simulink model "Vdc_Controller"  (R2022a)
settings: Solver=FixedStepAuto  StartTime=0.0  StopTime=TsimTime  FixedStep=Ts  MaxStep=Tsim*100  RelTol=1e-5
undefined symbols (not defined in the file): Avdc, Bvdc, IbuckSaturation, Kiv, Kpv, Ktv, Rdc, Ts
libraries: simulink x1
settings Model: Creator=MasterGnome  LastModifiedBy=MasterGnome
settings SolverCC: ZeroCrossAlgorithm=Adaptive
settings DataIOCC: SaveOutput=off  SaveTime=off
settings OptimizationCC: DefaultParameterBehavior=Inlined  EnhancedBackFolding=on  PassReuseOutputArgsAs=Individual arguments  ZeroExternalMemoryAtStartup=off  ZeroInternalMemoryAtStartup=off  OptimizeBlockOrder=speed  DifferentSizesBufferReuse=on  OptimizationCustomize=off  EfficientTunableParamExpr=on
settings DebuggingCC: IgnoredZcDiagnostic=none  ParameterTunabilityLossMsg=error  UnconnectedInputMsg=warning  UnconnectedOutputMsg=warning  UnconnectedLineMsg=warning
settings HardwareCC: ProdBitPerPointer=32  ProdBitPerSizeT=32  ProdBitPerPtrDiffT=32  ProdWordSize=32  ProdHWDeviceType=Intel->x86-32 (Windows32)  TargetBitPerPointer=64  TargetBitPerSizeT=64  TargetBitPerPtrDiffT=64  TargetLargestAtomicFloat=Float  TargetIntDivRoundTo=Zero  TargetEndianess=LittleEndian  TargetWordSize=64  TargetHWDeviceType=Intel->x86-64 (Windows64)
settings SFSimCC: MATLABDynamicMemAlloc=off
settings RTWCC: SystemTargetFile=ert.tlc  GenCodeOnly=on  TemplateMakefile=ert_default_tmf  DLArmComputeVersion=19.05
settings CodeAppCC: ForceParamTrailComments=on  IgnoreCustomStorageClasses=off  OperatorAnnotations=on  SimulinkDataObjDesc=on  SFDataObjDesc=on  InsertBlockDesc=on
settings ERTTargetCC: TargetLangStandard=C99 (ISO)  GenerateSampleERTMain=on  InlinedParameterPlacement=NonHierarchical  ERTCustomFileTemplate=example_file_process.tlc

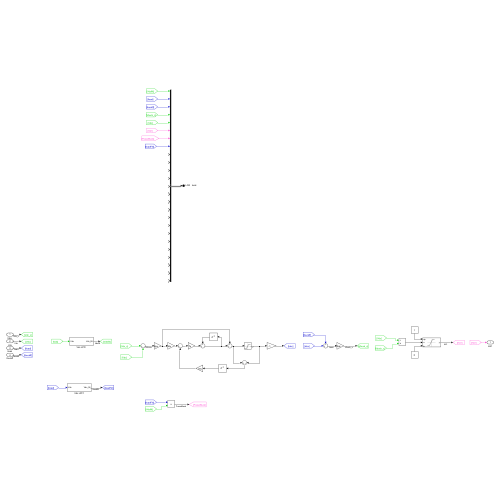
[thumbnail: Simulink's stored preview of the top-level diagram]
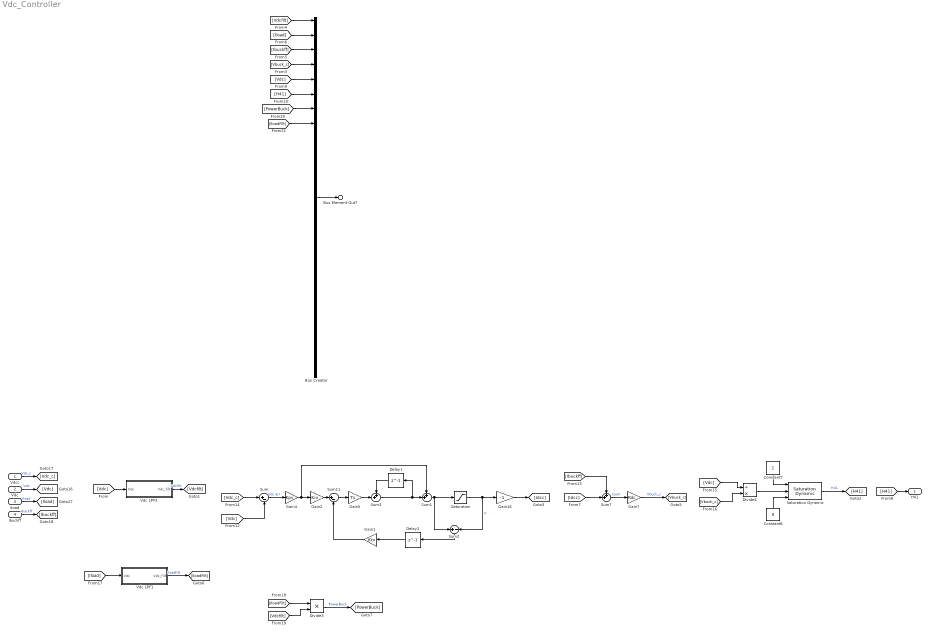
== system Vdc_Controller ==
  Vdcc : Inport  OutDataTypeStr=double  PortDimensions=1
  Vdc : Inport  Port=2  OutDataTypeStr=double  PortDimensions=1
  Iload : Inport  Port=3  OutDataTypeStr=double  PortDimensions=1
  Ibuckff : Inport  Port=4  OutDataTypeStr=double  PortDimensions=1
  Bus Creator : BusCreator  Inputs=25
  Constant6 : Constant  Value=0
  Constant7 : Constant
  Delay1 : Delay  DelayLength=1  SampleTime=Ts
  Delay2 : Delay  DelayLength=1  SampleTime=Ts
  Divide3 : Product  Inputs=**
  Divide4 : Product  Inputs=/*
  Gain1 : Gain  Gain=Ktv
  Gain16 : Gain  Gain=-1
  Gain2 : Gain  Gain=Kiv
  Gain4 : Gain  Gain=Kpv
  Gain5 : Gain  Gain=Ts
  Gain7 : Gain  Gain=Rdc
  Saturation : Saturate  UpperLimit=0  LowerLimit=-IbuckSaturation
  Saturation Dynamic : simulink/Discontinuities/Saturation Dynamic  OutMin=[]  OutMax=[]  OutDataTypeStr=Inherit: Same as second input  OutDataType=fixdt(1, 16)  OutScaling=2^-10  DoSatur=off
  Sum : Sum  Inputs=|+-
  Sum1 : Sum  Inputs=++|
  Sum11 : Sum  Inputs=|+-
  Sum2 : Sum  Inputs=+|-
  Sum3 : Sum  Inputs=++|
  Sum7 : Sum  Inputs=++|
  Vdc LPF1 : Subsystem
  Vdc LPF3 : Subsystem
  H41 : Outport  OutDataTypeStr=double  PortDimensions=1
  Bus Element Out7 : Outport  Port=2  PortName=LOG  Element=buck
  wires:
  Iload/1 -> [Iload]  "Iload"
  Vdc/1 -> [Vdc]  "Vdc"
  Vdcc/1 -> [Vdc_c]  "Vdc_c"
  Ibuckff/1 -> [Ibuckff]  "Ibuckff"
  Bus Creator/1 -> Bus Element Out7/1
  [Vdc] -> Vdc LPF3/1(Vdc)
  Vdc LPF3/1(Vdc_filt) -> [Vdcfilt]  "Vdcfilt"
  [Vdcfilt] -> Bus Creator/1
  [Iload] -> Bus Creator/2
  [Ibuckff] -> Bus Creator/3
  [Vbuck_c] -> Bus Creator/4
  [H41] -> H41/1
  [Vdc] -> Bus Creator/5
  [H41] -> Bus Creator/6
  Gain1/1 -> Sum11/2
  Gain4/1 -> Gain2/1, Sum1/1
  Gain5/1 -> Sum3/2
  Sum1/1 -> Sum2/1, Saturation/1
  Delay2/1 -> Gain1/1
  Sum7/1 -> Gain7/1  "Isum"
  Sum/1 -> Gain4/1  "Vdc err"
  [Ibuckff] -> Sum7/1
  [Idcc] -> Sum7/2
  Gain16/1 -> [Idcc]
  Gain7/1 -> [Vbuck_c]  "Vbuck_c"
  [Vdc] -> Sum/2
  Sum3/1 -> Sum1/2, Delay1/1
  Saturation/1 -> Gain16/1, Sum2/2  "I*"
  Delay1/1 -> Sum3/1
  [Vdc_c] -> Sum/1
  Sum11/1 -> Gain5/1
  Sum2/1 -> Delay2/1
  Gain2/1 -> Sum11/1
  Divide4/1 -> Saturation Dynamic/2
  Saturation Dynamic/1 -> [H41]  "H41"
  Constant6/1 -> Saturation Dynamic/3
  [Vdc] -> Divide4/1
  [Vbuck_c] -> Divide4/2
  Constant7/1 -> Saturation Dynamic/1
  [Iload] -> Vdc LPF1/1(Vdc)
  Vdc LPF1/1(Vdc_filt) -> [IloadFilt]  "Iloadfilt"
  [IloadFilt] -> Divide3/1
  [Vdcfilt] -> Divide3/2
  Divide3/1 -> [PowerBuck]  "PowerBuck"
  [PowerBuck] -> Bus Creator/7
  [IloadFilt] -> Bus Creator/8

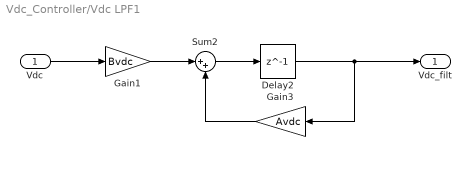
== system Vdc_Controller/Vdc LPF1 ==
  Vdc : Inport
  Delay2 : Delay  DelayLength=1  InitialCondition=0  SampleTime=Ts
  Gain1 : Gain  Gain=Bvdc
  Gain3 : Gain  Gain=Avdc
  Sum2 : Sum  Inputs=|++
  Vdc_filt : Outport
  wires:
  Vdc/1 -> Gain1/1
  Delay2/1 -> Vdc_filt/1, Gain3/1
  Sum2/1 -> Delay2/1
  Gain1/1 -> Sum2/1
  Gain3/1 -> Sum2/2

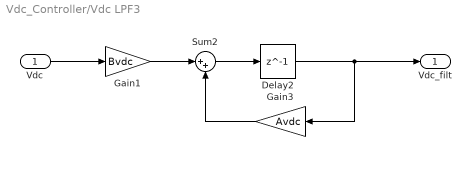
== system Vdc_Controller/Vdc LPF3 ==
  Vdc : Inport
  Delay2 : Delay  DelayLength=1  InitialCondition=0  SampleTime=Ts
  Gain1 : Gain  Gain=Bvdc
  Gain3 : Gain  Gain=Avdc
  Sum2 : Sum  Inputs=|++
  Vdc_filt : Outport
  wires:
  Vdc/1 -> Gain1/1
  Delay2/1 -> Vdc_filt/1, Gain3/1
  Sum2/1 -> Delay2/1
  Gain1/1 -> Sum2/1
  Gain3/1 -> Sum2/2
